simulink model "unityVPC"  (R2021a)
settings: Solver=FixedStepAuto  StartTime=0.0  StopTime=inf  FixedStep=0.02  RelTol=1e-3
undefined symbols (not defined in the file): alpha, Angular, gd, Kc, Linear, ros_freq, Rx, Ry, Rz, T, var_max, X, Y, Z
libraries: simlib_vpc_coremath x26, robotlib x20, simlib_vpc_basic x10, dspmtrx3 x4, simlib_vpc_gp x3
settings Model: EnablePacing=on  OrderedModelArguments=off  Creator=marco  LastModifiedBy=marco
settings DebuggingCC: AlgebraicLoopMsg=none

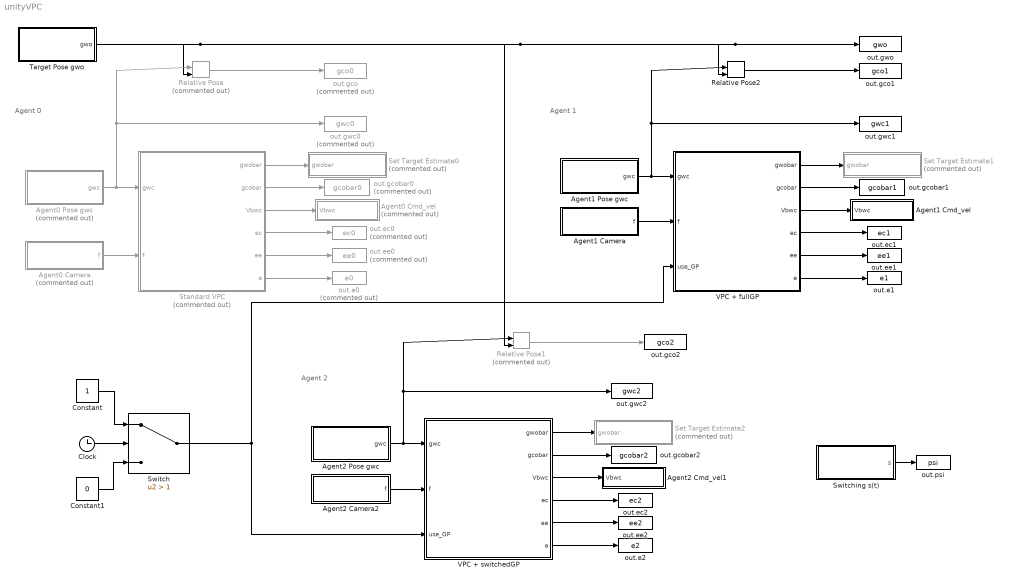
== system unityVPC ==
  note: Agent 0
  note: Agent 1
  note: Agent 2
  Agent0 Camera : Subsystem  Commented=on
  Agent0 Cmd_vel : Subsystem  Commented=on
  Agent0 Pose gwc : Subsystem  Commented=on
  Agent1 Camera : Subsystem
  Agent1 Cmd_vel : Subsystem
  Agent1 Pose gwc : Subsystem
  Agent2 Camera2 : Subsystem
  Agent2 Cmd_vel1 : Subsystem
  Agent2 Pose gwc : Subsystem
  Clock : Clock
  Constant : Constant
  Constant1 : Constant  Value=0
  Relative Pose : simlib_vpc_coremath/Relative Pose  Commented=on
      settings: SourceProductName=VPC Library
  Relative Pose1 : simlib_vpc_coremath/Relative Pose  Commented=on
      settings: SourceProductName=VPC Library
  Relative Pose2 : simlib_vpc_coremath/Relative Pose
      settings: SourceProductName=VPC Library
  Set Target Estimate0 : Subsystem  Commented=on
  Set Target Estimate1 : Subsystem  Commented=on
  Set Target Estimate2 : Subsystem  Commented=on
  Standard VPC : Subsystem  Commented=on
      mask Display:
      | disp('VPC without GP','texmode','on')
      | 
      | % Label ports
      | port_label('input',1,'g_{wc}','texmode','on')
      | port_label('input',2,'f','texmode','on')
      | port_label('output',1,'g_{wo,bar}','texmode','on')
      | port_label('output',2,'gco,bar','texmode','on')
      | port_label('output',3,'V^b_{wc}','texmode','on')
      | port_label('output',4,'ec','texmode','on')
      | port_label('output',5,'ee','texmode','on')
      | port_label('output',6,'e','texmode','on')
  Switch : Switch  Criteria=u2 > Threshold  Threshold=1
  Switching s(t) : Subsystem
  Target Pose gwo : Subsystem
  VPC + fullGP : Subsystem
      mask Display:
      | disp('VPC + fullGP','texmode','on')
      | 
      | % Label ports
      | port_label('input',1,'g_{wc}','texmode','on')
      | port_label('input',2,'f','texmode','on')
      | port_label('output',1,'g_{wo,bar}','texmode','on')
      | port_label('output',2,'gco,bar','texmode','on')
      | port_label('output',3,'V^b_{wc}','texmode','on')
      | port_label('output',4,'ec','texmode','on')
      | port_label('output',5,'ee','texmode','on')
      | port_label('output',6,'e','texmode','on')
  VPC + switchedGP : Subsystem
      mask Display:
      | disp('VPC + switchedGP','texmode','on')
      | 
      | % Label ports
      | port_label('input',1,'g_{wc}','texmode','on')
      | port_label('input',2,'f','texmode','on')
      | port_label('output',1,'g_{wo,bar}','texmode','on')
      | port_label('output',2,'gco,bar','texmode','on')
      | port_label('output',3,'V^b_{wc}','texmode','on')
      | port_label('output',4,'ec','texmode','on')
      | port_label('output',5,'ee','texmode','on')
      | port_label('output',6,'e','texmode','on')
  out.e0 : ToWorkspace  Commented=on  VariableName=e0  SaveFormat=Structure With Time  SampleTime=-1
  out.e1 : ToWorkspace  VariableName=e1  SaveFormat=Structure With Time  SampleTime=-1
  out.e2 : ToWorkspace  VariableName=e2  SaveFormat=Structure With Time  SampleTime=-1
  out.ec0 : ToWorkspace  Commented=on  VariableName=ec0  SaveFormat=Structure With Time  SampleTime=-1
  out.ec1 : ToWorkspace  VariableName=ec1  SaveFormat=Structure With Time  SampleTime=-1
  out.ec2 : ToWorkspace  VariableName=ec2  SaveFormat=Structure With Time  SampleTime=-1
  out.ee0 : ToWorkspace  Commented=on  VariableName=ee0  SaveFormat=Structure With Time  SampleTime=-1
  out.ee1 : ToWorkspace  VariableName=ee1  SaveFormat=Structure With Time  SampleTime=-1
  out.ee2 : ToWorkspace  VariableName=ee2  SaveFormat=Structure With Time  SampleTime=-1
  out.gco : ToWorkspace  Commented=on  VariableName=gco0  SaveFormat=Structure With Time  SampleTime=-1
  out.gco1 : ToWorkspace  VariableName=gco1  SaveFormat=Structure With Time  SampleTime=-1
  out.gco2 : ToWorkspace  VariableName=gco2  SaveFormat=Structure With Time  SampleTime=-1
  out.gcobar0 : ToWorkspace  Commented=on  VariableName=gcobar0  SaveFormat=Structure With Time  SampleTime=-1
  out.gcobar1 : ToWorkspace  VariableName=gcobar1  SaveFormat=Structure With Time  SampleTime=-1
  out.gcobar2 : ToWorkspace  VariableName=gcobar2  SaveFormat=Structure With Time  SampleTime=-1
  out.gwc0 : ToWorkspace  Commented=on  VariableName=gwc0  SaveFormat=Structure With Time  SampleTime=-1
  out.gwc1 : ToWorkspace  VariableName=gwc1  SaveFormat=Structure With Time  SampleTime=-1
  out.gwc2 : ToWorkspace  VariableName=gwc2  SaveFormat=Structure With Time  SampleTime=-1
  out.gwo : ToWorkspace  VariableName=gwo  SaveFormat=Structure With Time  SampleTime=-1
  out.psi : ToWorkspace  VariableName=psi  SaveFormat=Structure With Time  SampleTime=-1
  wires:
  Standard VPC/1(gwobar) -> Set Target Estimate0/1(gwobar)
  Agent0 Camera/1(f) -> Standard VPC/2(f)
  Relative Pose/1 -> out.gco/1
  Target Pose gwo/1(gwo) -> out.gwo/1, Relative Pose2/2, Relative Pose1/2, Relative Pose/2
  Agent0 Pose gwc/1(gwc) -> Relative Pose/1, out.gwc0/1, Standard VPC/1(gwc)
  Standard VPC/4(ec) -> out.ec0/1
  Standard VPC/5(ee) -> out.ee0/1
  Standard VPC/6(e) -> out.e0/1
  Standard VPC/2(gcobar) -> out.gcobar0/1
  Standard VPC/3(Vbwc) -> Agent0 Cmd_vel/1(Vbwc)
  Relative Pose1/1 -> out.gco2/1
  VPC + fullGP/4(ec) -> out.ec1/1
  VPC + fullGP/2(gcobar) -> out.gcobar1/1
  VPC + fullGP/5(ee) -> out.ee1/1
  VPC + fullGP/3(Vbwc) -> Agent1 Cmd_vel/1(Vbwc)
  Agent1 Pose gwc/1(gwc) -> Relative Pose2/1, out.gwc1/1, VPC + fullGP/1(gwc)
  VPC + fullGP/1(gwobar) -> Set Target Estimate1/1(gwobar)
  VPC + fullGP/6(e) -> out.e1/1
  Agent1 Camera/1(f) -> VPC + fullGP/2(f)
  Relative Pose2/1 -> out.gco1/1
  VPC + switchedGP/4(ec) -> out.ec2/1
  Agent2 Pose gwc/1(gwc) -> Relative Pose1/1, out.gwc2/1, VPC + switchedGP/1(gwc)
  VPC + switchedGP/2(gcobar) -> out.gcobar2/1
  Agent2 Camera2/1(f) -> VPC + switchedGP/2(f)
  VPC + switchedGP/5(ee) -> out.ee2/1
  VPC + switchedGP/1(gwobar) -> Set Target Estimate2/1(gwobar)
  VPC + switchedGP/3(Vbwc) -> Agent2 Cmd_vel1/1(Vbwc)
  VPC + switchedGP/6(e) -> out.e2/1
  Switching s(t)/1(s) -> out.psi/1
  Constant/1 -> Switch/1
  Constant1/1 -> Switch/3
  Switch/1 -> VPC + switchedGP/3(use_GP), VPC + fullGP/3(use_GP)
  Clock/1 -> Switch/2

== system unityVPC/Agent0 Camera ==
  Bus Selector1 : BusSelector  OutputSignals=Fp1X,Fp1Y,Fp2X,Fp2Y,Fp3X,Fp3Y,Fp4X,Fp4Y
  Data Type Conversion : DataTypeConversion  OutDataTypeStr=double
  Subscribe1 : robotlib/Subscribe  topicSource=Specify your own  topic=/agent0_vcam  messageType=custom_msgs/VisMea  SampleTime=-1  legacyBusStruct=off  messageQueueLength=1
  Terminator1 : Terminator
  Vector Concatenate : Concatenate  NumInputs=8
  f : Outport
  wires:
  Bus Selector1/4 -> Vector Concatenate/4  "<Fp2Y>"
  Data Type Conversion/1 -> f/1
  Bus Selector1/2 -> Vector Concatenate/2  "<Fp1Y>"
  Bus Selector1/3 -> Vector Concatenate/3  "<Fp2X>"
  Vector Concatenate/1 -> Data Type Conversion/1
  Subscribe1/1 -> Terminator1/1
  Bus Selector1/5 -> Vector Concatenate/5  "<Fp3X>"
  Bus Selector1/1 -> Vector Concatenate/1  "<Fp1X>"
  Subscribe1/2 -> Bus Selector1/1
  Bus Selector1/7 -> Vector Concatenate/7  "<Fp4X>"
  Bus Selector1/6 -> Vector Concatenate/6  "<Fp3Y>"
  Bus Selector1/8 -> Vector Concatenate/8  "<Fp4Y>"

== system unityVPC/Agent0 Cmd_vel ==
  note: Update estimate in Unity simulation
  Vbwc : Inport
  Blank Message : robotlib/Blank Message  messageClass=Message  entityType=geometry_msgs/Twist  messageType=geometry_msgs/Twist  SampleTime=inf  legacyBusStruct=off
  Bus Assignment1 : BusAssignment  AssignedSignals=Linear.X,Linear.Y,Linear.Z,Angular.X,Angular.Y,Angular.Z
  Demux1 : Demux  Outputs=6
  Gain : Gain  Gain=-1
  Gain1 : Gain  Gain=-1
  Gain2 : Gain  Gain=-1
  Publish : robotlib/Publish  topicSource=Specify your own  topic=/agent0_Vbwc  messageType=geometry_msgs/Twist  legacyBusStruct=off  messageQueueLength=1
  Rate Transition : RateTransition  Commented=through  OutPortSampleTime=1/ros_freq
  wires:
  Blank Message/1 -> Bus Assignment1/1
  Bus Assignment1/1 -> Publish/1
  Demux1/1 -> Bus Assignment1/2
  Demux1/4 -> Gain/1
  Vbwc/1 -> Rate Transition/1
  Demux1/5 -> Gain2/1
  Demux1/2 -> Bus Assignment1/4
  Demux1/3 -> Bus Assignment1/3
  Demux1/6 -> Gain1/1
  Gain/1 -> Bus Assignment1/5
  Gain1/1 -> Bus Assignment1/6
  Gain2/1 -> Bus Assignment1/7
  Rate Transition/1 -> Demux1/1

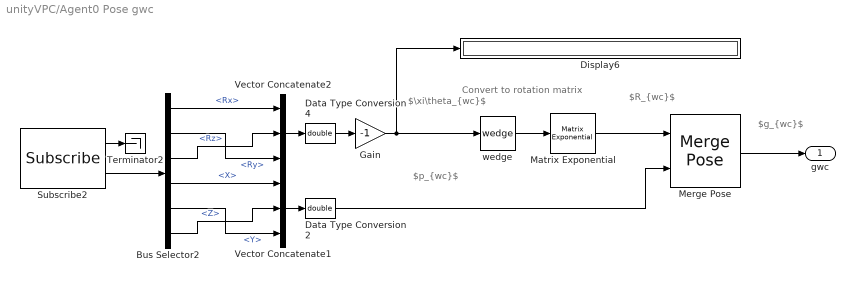
== system unityVPC/Agent0 Pose gwc ==
  note: $g_{wc}$
  note: $R_{wc}$
  note: $p_{wc}$
  note: $\xi\theta_{wc}$
  note: Convert to rotation matrix
  Bus Selector2 : BusSelector  OutputSignals=Rx,Ry,Rz,X,Y,Z
  Data Type Conversion2 : DataTypeConversion  OutDataTypeStr=double
  Data Type Conversion4 : DataTypeConversion  OutDataTypeStr=double
  Display6 : Display
  Gain : Gain  Gain=-1
  Matrix Exponential : dspmtrx3/Matrix Exponential
      settings: SourceProductBaseCode=DS
  Merge Pose : simlib_vpc_coremath/Merge Pose
      settings: SourceProductName=VPC Library
  Subscribe2 : robotlib/Subscribe  topicSource=Specify your own  topic=/agent0_pose  messageType=custom_msgs/PosRot  SampleTime=-1  legacyBusStruct=off  messageQueueLength=1
  Terminator2 : Terminator
  Vector Concatenate1 : Concatenate  NumInputs=3
  Vector Concatenate2 : Concatenate  NumInputs=3
  wedge : simlib_vpc_coremath/wedge
      settings: SourceProductName=VPC Library
  gwc : Outport
  wires:
  Vector Concatenate2/1 -> Data Type Conversion4/1
  Subscribe2/1 -> Terminator2/1
  Matrix Exponential/1 -> Merge Pose/1
  Vector Concatenate1/1 -> Data Type Conversion2/1
  Data Type Conversion2/1 -> Merge Pose/2
  Subscribe2/2 -> Bus Selector2/1
  Bus Selector2/1 -> Vector Concatenate2/1  "<Rx>"
  Bus Selector2/4 -> Vector Concatenate1/1  "<X>"
  Data Type Conversion4/1 -> Gain/1
  wedge/1 -> Matrix Exponential/1
  Bus Selector2/2 -> Vector Concatenate2/3  "<Ry>"
  Merge Pose/1 -> gwc/1
  Bus Selector2/5 -> Vector Concatenate1/3  "<Y>"
  Bus Selector2/6 -> Vector Concatenate1/2  "<Z>"
  Bus Selector2/3 -> Vector Concatenate2/2  "<Rz>"
  Gain/1 -> Display6/1, wedge/1

== system unityVPC/Agent1 Camera ==
  Bus Selector1 : BusSelector  OutputSignals=Fp1X,Fp1Y,Fp2X,Fp2Y,Fp3X,Fp3Y,Fp4X,Fp4Y
  Data Type Conversion : DataTypeConversion  OutDataTypeStr=double
  Subscribe1 : robotlib/Subscribe  topicSource=Select from ROS network  topic=/agent1_vcam  messageType=custom_msgs/VisMea  SampleTime=-1  legacyBusStruct=off  messageQueueLength=1
  Terminator1 : Terminator
  Vector Concatenate : Concatenate  NumInputs=8
  f : Outport
  wires:
  Bus Selector1/4 -> Vector Concatenate/4  "<Fp2Y>"
  Data Type Conversion/1 -> f/1
  Bus Selector1/2 -> Vector Concatenate/2  "<Fp1Y>"
  Bus Selector1/3 -> Vector Concatenate/3  "<Fp2X>"
  Vector Concatenate/1 -> Data Type Conversion/1
  Subscribe1/1 -> Terminator1/1
  Bus Selector1/5 -> Vector Concatenate/5  "<Fp3X>"
  Bus Selector1/1 -> Vector Concatenate/1  "<Fp1X>"
  Subscribe1/2 -> Bus Selector1/1
  Bus Selector1/7 -> Vector Concatenate/7  "<Fp4X>"
  Bus Selector1/6 -> Vector Concatenate/6  "<Fp3Y>"
  Bus Selector1/8 -> Vector Concatenate/8  "<Fp4Y>"

== system unityVPC/Agent1 Cmd_vel ==
  note: Update estimate in Unity simulation
  Vbwc : Inport
  Blank Message : robotlib/Blank Message  messageClass=Message  entityType=geometry_msgs/Twist  messageType=geometry_msgs/Twist  SampleTime=inf  legacyBusStruct=off
  Bus Assignment1 : BusAssignment  AssignedSignals=Linear.X,Linear.Y,Linear.Z,Angular.X,Angular.Y,Angular.Z
  Demux1 : Demux  Outputs=6
  Gain : Gain  Gain=-1
  Gain1 : Gain  Gain=-1
  Gain2 : Gain  Gain=-1
  Publish : robotlib/Publish  topicSource=Select from ROS network  topic=/agent1_Vbwc  messageType=geometry_msgs/Twist  legacyBusStruct=off  messageQueueLength=1
  Rate Transition : RateTransition  OutPortSampleTime=1/ros_freq
  wires:
  Blank Message/1 -> Bus Assignment1/1
  Bus Assignment1/1 -> Publish/1
  Demux1/1 -> Bus Assignment1/2
  Demux1/4 -> Gain/1
  Vbwc/1 -> Rate Transition/1
  Demux1/5 -> Gain2/1
  Demux1/2 -> Bus Assignment1/4
  Demux1/3 -> Bus Assignment1/3
  Demux1/6 -> Gain1/1
  Gain/1 -> Bus Assignment1/5
  Gain1/1 -> Bus Assignment1/6
  Gain2/1 -> Bus Assignment1/7
  Rate Transition/1 -> Demux1/1

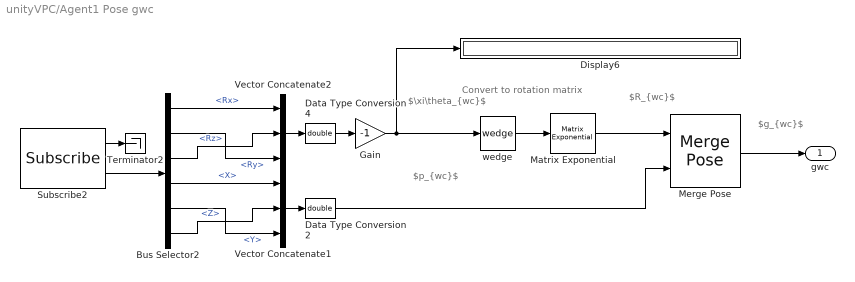
== system unityVPC/Agent1 Pose gwc ==
  note: $g_{wc}$
  note: $R_{wc}$
  note: $p_{wc}$
  note: $\xi\theta_{wc}$
  note: Convert to rotation matrix
  Bus Selector2 : BusSelector  OutputSignals=Rx,Ry,Rz,X,Y,Z
  Data Type Conversion2 : DataTypeConversion  OutDataTypeStr=double
  Data Type Conversion4 : DataTypeConversion  OutDataTypeStr=double
  Display6 : Display
  Gain : Gain  Gain=-1
  Matrix Exponential : dspmtrx3/Matrix Exponential
      settings: SourceProductBaseCode=DS
  Merge Pose : simlib_vpc_coremath/Merge Pose
      settings: SourceProductName=VPC Library
  Subscribe2 : robotlib/Subscribe  topicSource=Select from ROS network  topic=/agent1_pose  messageType=custom_msgs/PosRot  SampleTime=-1  legacyBusStruct=off  messageQueueLength=1
  Terminator2 : Terminator
  Vector Concatenate1 : Concatenate  NumInputs=3
  Vector Concatenate2 : Concatenate  NumInputs=3
  wedge : simlib_vpc_coremath/wedge
      settings: SourceProductName=VPC Library
  gwc : Outport
  wires:
  Vector Concatenate2/1 -> Data Type Conversion4/1
  Subscribe2/1 -> Terminator2/1
  Matrix Exponential/1 -> Merge Pose/1
  Vector Concatenate1/1 -> Data Type Conversion2/1
  Data Type Conversion2/1 -> Merge Pose/2
  Subscribe2/2 -> Bus Selector2/1
  Bus Selector2/1 -> Vector Concatenate2/1  "<Rx>"
  Bus Selector2/4 -> Vector Concatenate1/1  "<X>"
  Data Type Conversion4/1 -> Gain/1
  wedge/1 -> Matrix Exponential/1
  Bus Selector2/2 -> Vector Concatenate2/3  "<Ry>"
  Merge Pose/1 -> gwc/1
  Bus Selector2/5 -> Vector Concatenate1/3  "<Y>"
  Bus Selector2/6 -> Vector Concatenate1/2  "<Z>"
  Bus Selector2/3 -> Vector Concatenate2/2  "<Rz>"
  Gain/1 -> Display6/1, wedge/1

== system unityVPC/Agent2 Camera2 ==
  Bus Selector1 : BusSelector  OutputSignals=Fp1X,Fp1Y,Fp2X,Fp2Y,Fp3X,Fp3Y,Fp4X,Fp4Y
  Data Type Conversion : DataTypeConversion  OutDataTypeStr=double
  Subscribe1 : robotlib/Subscribe  topicSource=Specify your own  topic=/agent2_vcam  messageType=custom_msgs/VisMea  SampleTime=-1  legacyBusStruct=off  messageQueueLength=1
  Terminator1 : Terminator
  Vector Concatenate : Concatenate  NumInputs=8
  f : Outport
  wires:
  Bus Selector1/4 -> Vector Concatenate/4  "<Fp2Y>"
  Data Type Conversion/1 -> f/1
  Bus Selector1/2 -> Vector Concatenate/2  "<Fp1Y>"
  Bus Selector1/3 -> Vector Concatenate/3  "<Fp2X>"
  Vector Concatenate/1 -> Data Type Conversion/1
  Subscribe1/1 -> Terminator1/1
  Bus Selector1/5 -> Vector Concatenate/5  "<Fp3X>"
  Bus Selector1/1 -> Vector Concatenate/1  "<Fp1X>"
  Subscribe1/2 -> Bus Selector1/1
  Bus Selector1/7 -> Vector Concatenate/7  "<Fp4X>"
  Bus Selector1/6 -> Vector Concatenate/6  "<Fp3Y>"
  Bus Selector1/8 -> Vector Concatenate/8  "<Fp4Y>"

== system unityVPC/Agent2 Cmd_vel1 ==
  note: Update estimate in Unity simulation
  Vbwc : Inport
  Blank Message : robotlib/Blank Message  messageClass=Message  entityType=geometry_msgs/Twist  messageType=geometry_msgs/Twist  SampleTime=inf  legacyBusStruct=off
  Bus Assignment1 : BusAssignment  AssignedSignals=Linear.X,Linear.Y,Linear.Z,Angular.X,Angular.Y,Angular.Z
  Demux1 : Demux  Outputs=6
  Gain : Gain  Gain=-1
  Gain1 : Gain  Gain=-1
  Gain2 : Gain  Gain=-1
  Publish : robotlib/Publish  topicSource=Specify your own  topic=/agent2_Vbwc  messageType=geometry_msgs/Twist  legacyBusStruct=off  messageQueueLength=1
  Rate Transition : RateTransition  OutPortSampleTime=1/ros_freq
  wires:
  Blank Message/1 -> Bus Assignment1/1
  Bus Assignment1/1 -> Publish/1
  Demux1/1 -> Bus Assignment1/2
  Demux1/4 -> Gain/1
  Vbwc/1 -> Rate Transition/1
  Demux1/5 -> Gain2/1
  Demux1/2 -> Bus Assignment1/4
  Demux1/3 -> Bus Assignment1/3
  Demux1/6 -> Gain1/1
  Gain/1 -> Bus Assignment1/5
  Gain1/1 -> Bus Assignment1/6
  Gain2/1 -> Bus Assignment1/7
  Rate Transition/1 -> Demux1/1

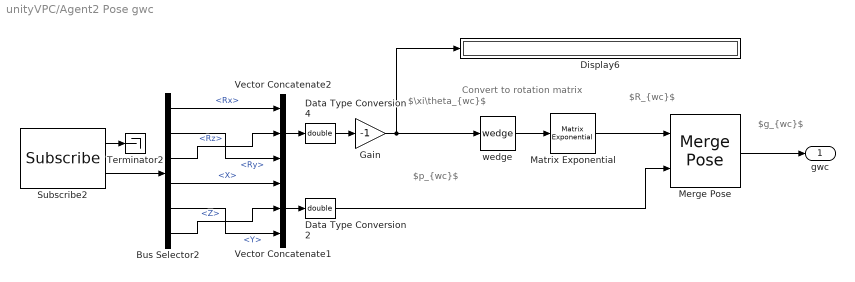
== system unityVPC/Agent2 Pose gwc ==
  note: $g_{wc}$
  note: $R_{wc}$
  note: $p_{wc}$
  note: $\xi\theta_{wc}$
  note: Convert to rotation matrix
  Bus Selector2 : BusSelector  OutputSignals=Rx,Ry,Rz,X,Y,Z
  Data Type Conversion2 : DataTypeConversion  OutDataTypeStr=double
  Data Type Conversion4 : DataTypeConversion  OutDataTypeStr=double
  Display6 : Display
  Gain : Gain  Gain=-1
  Matrix Exponential : dspmtrx3/Matrix Exponential
      settings: SourceProductBaseCode=DS
  Merge Pose : simlib_vpc_coremath/Merge Pose
      settings: SourceProductName=VPC Library
  Subscribe2 : robotlib/Subscribe  topicSource=Specify your own  topic=/agent2_pose  messageType=custom_msgs/PosRot  SampleTime=-1  legacyBusStruct=off  messageQueueLength=1
  Terminator2 : Terminator
  Vector Concatenate1 : Concatenate  NumInputs=3
  Vector Concatenate2 : Concatenate  NumInputs=3
  wedge : simlib_vpc_coremath/wedge
      settings: SourceProductName=VPC Library
  gwc : Outport
  wires:
  Vector Concatenate2/1 -> Data Type Conversion4/1
  Subscribe2/1 -> Terminator2/1
  Matrix Exponential/1 -> Merge Pose/1
  Vector Concatenate1/1 -> Data Type Conversion2/1
  Data Type Conversion2/1 -> Merge Pose/2
  Subscribe2/2 -> Bus Selector2/1
  Bus Selector2/1 -> Vector Concatenate2/1  "<Rx>"
  Bus Selector2/4 -> Vector Concatenate1/1  "<X>"
  Data Type Conversion4/1 -> Gain/1
  wedge/1 -> Matrix Exponential/1
  Bus Selector2/2 -> Vector Concatenate2/3  "<Ry>"
  Merge Pose/1 -> gwc/1
  Bus Selector2/5 -> Vector Concatenate1/3  "<Y>"
  Bus Selector2/6 -> Vector Concatenate1/2  "<Z>"
  Bus Selector2/3 -> Vector Concatenate2/2  "<Rz>"
  Gain/1 -> Display6/1, wedge/1

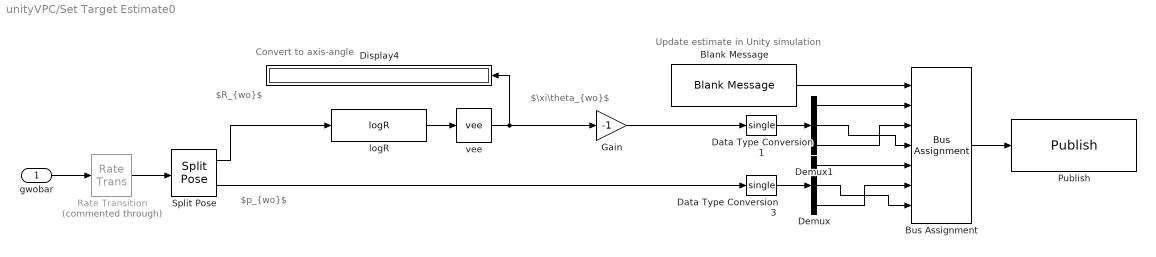
== system unityVPC/Set Target Estimate0 ==
  note: $\xi\theta_{wo}$
  note: $p_{wo}$
  note: Convert to axis-angle
  note: $R_{wo}$
  note: Update estimate in Unity simulation
  gwobar : Inport
  Blank Message : robotlib/Blank Message  messageClass=Message  entityType=custom_msgs/PosRot  messageType=custom_msgs/PosRot  SampleTime=inf  legacyBusStruct=off
  Bus Assignment : BusAssignment  AssignedSignals=Rx,Ry,Rz,X,Y,Z
  Data Type Conversion1 : DataTypeConversion  OutDataTypeStr=single
  Data Type Conversion3 : DataTypeConversion  OutDataTypeStr=single
  Demux : Demux  Outputs=3
  Demux1 : Demux  Outputs=3
  Display4 : Display
  Gain : Gain  Gain=-1
  Publish : robotlib/Publish  topicSource=Select from ROS network  topic=/estim_pose  messageType=custom_msgs/PosRot  legacyBusStruct=off  messageQueueLength=1
  Rate Transition : RateTransition  Commented=through  OutPortSampleTime=1/ros_freq
  Split Pose : simlib_vpc_coremath/Split Pose
      settings: SourceProductName=VPC Library
  logR : simlib_vpc_coremath/logR
      settings: SourceProductName=VPC Library
  vee : simlib_vpc_coremath/vee
      settings: SourceProductName=VPC Library
  wires:
  Bus Assignment/1 -> Publish/1
  Demux1/1 -> Bus Assignment/2
  Data Type Conversion1/1 -> Demux1/1
  Demux1/2 -> Bus Assignment/4
  vee/1 -> Gain/1, Display4/1
  Split Pose/1 -> logR/1
  Demux/3 -> Bus Assignment/6
  Blank Message/1 -> Bus Assignment/1
  Demux1/3 -> Bus Assignment/3
  Split Pose/2 -> Data Type Conversion3/1
  Demux/1 -> Bus Assignment/5
  logR/1 -> vee/1
  Data Type Conversion3/1 -> Demux/1
  Demux/2 -> Bus Assignment/7
  gwobar/1 -> Rate Transition/1
  Gain/1 -> Data Type Conversion1/1
  Rate Transition/1 -> Split Pose/1

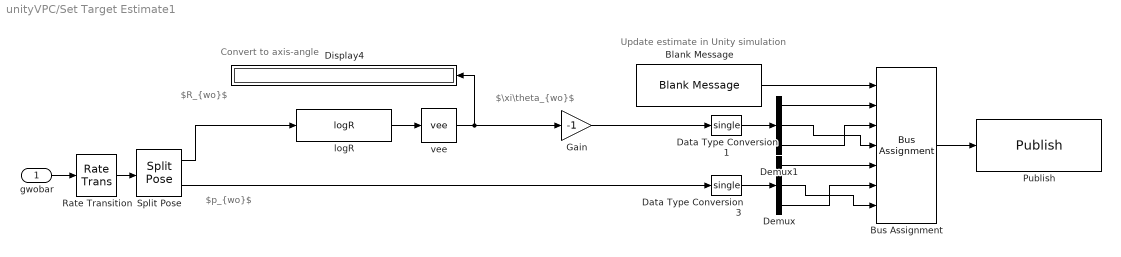
== system unityVPC/Set Target Estimate1 ==
  note: $\xi\theta_{wo}$
  note: $p_{wo}$
  note: Convert to axis-angle
  note: $R_{wo}$
  note: Update estimate in Unity simulation
  gwobar : Inport
  Blank Message : robotlib/Blank Message  messageClass=Message  entityType=custom_msgs/PosRot  messageType=custom_msgs/PosRot  SampleTime=inf  legacyBusStruct=off
  Bus Assignment : BusAssignment  AssignedSignals=Rx,Ry,Rz,X,Y,Z
  Data Type Conversion1 : DataTypeConversion  OutDataTypeStr=single
  Data Type Conversion3 : DataTypeConversion  OutDataTypeStr=single
  Demux : Demux  Outputs=3
  Demux1 : Demux  Outputs=3
  Display4 : Display
  Gain : Gain  Gain=-1
  Publish : robotlib/Publish  topicSource=Select from ROS network  topic=/estim_pose  messageType=custom_msgs/PosRot  legacyBusStruct=off  messageQueueLength=1
  Rate Transition : RateTransition  OutPortSampleTime=1/ros_freq
  Split Pose : simlib_vpc_coremath/Split Pose
      settings: SourceProductName=VPC Library
  logR : simlib_vpc_coremath/logR
      settings: SourceProductName=VPC Library
  vee : simlib_vpc_coremath/vee
      settings: SourceProductName=VPC Library
  wires:
  Bus Assignment/1 -> Publish/1
  Demux1/1 -> Bus Assignment/2
  Data Type Conversion1/1 -> Demux1/1
  Demux1/2 -> Bus Assignment/4
  vee/1 -> Gain/1, Display4/1
  Split Pose/1 -> logR/1
  Demux/3 -> Bus Assignment/6
  Blank Message/1 -> Bus Assignment/1
  Demux1/3 -> Bus Assignment/3
  Split Pose/2 -> Data Type Conversion3/1
  Demux/1 -> Bus Assignment/5
  logR/1 -> vee/1
  Data Type Conversion3/1 -> Demux/1
  Demux/2 -> Bus Assignment/7
  gwobar/1 -> Rate Transition/1
  Gain/1 -> Data Type Conversion1/1
  Rate Transition/1 -> Split Pose/1

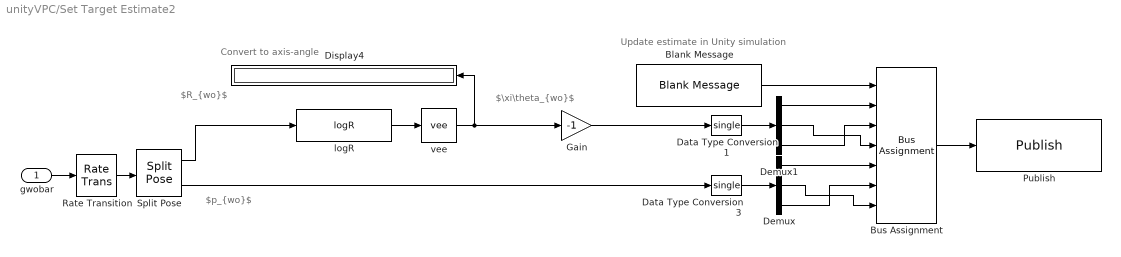
== system unityVPC/Set Target Estimate2 ==
  note: $\xi\theta_{wo}$
  note: $p_{wo}$
  note: Convert to axis-angle
  note: $R_{wo}$
  note: Update estimate in Unity simulation
  gwobar : Inport
  Blank Message : robotlib/Blank Message  messageClass=Message  entityType=custom_msgs/PosRot  messageType=custom_msgs/PosRot  SampleTime=inf  legacyBusStruct=off
  Bus Assignment : BusAssignment  AssignedSignals=Rx,Ry,Rz,X,Y,Z
  Data Type Conversion1 : DataTypeConversion  OutDataTypeStr=single
  Data Type Conversion3 : DataTypeConversion  OutDataTypeStr=single
  Demux : Demux  Outputs=3
  Demux1 : Demux  Outputs=3
  Display4 : Display
  Gain : Gain  Gain=-1
  Publish : robotlib/Publish  topicSource=Select from ROS network  topic=/estim_pose  messageType=custom_msgs/PosRot  legacyBusStruct=off  messageQueueLength=1
  Rate Transition : RateTransition  OutPortSampleTime=1/ros_freq
  Split Pose : simlib_vpc_coremath/Split Pose
      settings: SourceProductName=VPC Library
  logR : simlib_vpc_coremath/logR
      settings: SourceProductName=VPC Library
  vee : simlib_vpc_coremath/vee
      settings: SourceProductName=VPC Library
  wires:
  Bus Assignment/1 -> Publish/1
  Demux1/1 -> Bus Assignment/2
  Data Type Conversion1/1 -> Demux1/1
  Demux1/2 -> Bus Assignment/4
  vee/1 -> Gain/1, Display4/1
  Split Pose/1 -> logR/1
  Demux/3 -> Bus Assignment/6
  Blank Message/1 -> Bus Assignment/1
  Demux1/3 -> Bus Assignment/3
  Split Pose/2 -> Data Type Conversion3/1
  Demux/1 -> Bus Assignment/5
  logR/1 -> vee/1
  Data Type Conversion3/1 -> Demux/1
  Demux/2 -> Bus Assignment/7
  gwobar/1 -> Rate Transition/1
  Gain/1 -> Data Type Conversion1/1
  Rate Transition/1 -> Split Pose/1

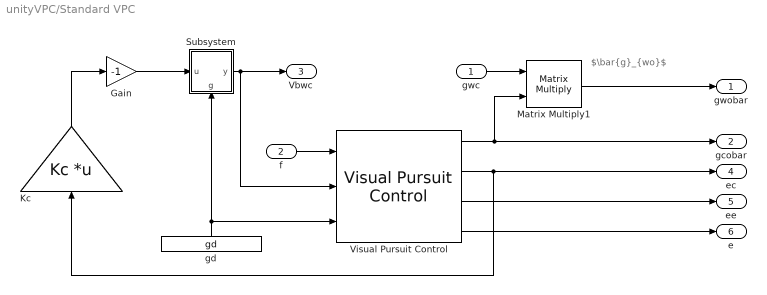
== system unityVPC/Standard VPC ==
  note: $\bar{g}_{wo}$
  gwc : Inport
  f : Inport  Port=2
  Gain : Gain  Gain=-1
  Kc : Gain  Gain=Kc  Multiplication=Matrix(K*u) (u vector)
  Matrix Multiply1 : Product  Multiplication=Matrix(*)
  Subsystem : Subsystem
      settings: PortSchema="{\"entries\":[{\"content\":{\"sides\":[{\"content\":{\"connectorIds\":[\"In1\"]},\"type\":\"ConnectorPlacement.EquallySpacedRectSide\",\"uuid\":\"72e68008-5c4a-43a9-a560-64c6a31a0c08\"},{\"content\":{\"connectorIds\":[\"Out1\"],\"side\":\"RIGHT\"},\"type\":\"ConnectorPlacement.EquallySpacedRectSide\",\"uuid\":\"da07f5ff-2b2c-4c55-a2f2-34e133777503\"},{\"content\":{\"connectorIds\":[],\"side\":\"TOP\"},\"type\":\"ConnectorPlacement.EquallySpacedRectSide\",\"uuid\":\"6d174428-4364-4e89-aba7-4e9864808ab5\"},{\"content\":{\"connectorIds\":[\"In2\"],\"side\":\"BOTTOM\"},\"type\":\"ConnectorPlacement.EquallySpacedRectSide\",\"uuid\":\"f9633104-9c11-4d21-90a7-e0f886d9e92d\"},{\"content\":{\"connectorIds\":[],\"side\":\"HIDDEN\"},\"type\":\"ConnectorPlacement.EquallySpacedRectSide\",\"uuid\":\"662f08ae-9279-4a4f-85ea-81d97ead27d9\"}]},\"type\":\"ConnectorPlacement.EquallySpacedConnector\",\"uuid\":\"f3cd156c-cccd-47c6-b81c-6113f78efd58\"}],\"packageUris\":[\"http://schema.mathworks.com/mf0/Connector/R2020b\"],\"version\":\"1.0\"}"
      mask Display:
      | % Glitch in Matlab: If you define a line whose starting point and end point
      | % is equal, then the entire mask block is plotted in bold
      | plot([0,0],[0,0])
      | 
      | % Draw box
      | indent = 0.3;
      | ang=[0:0.2:pi/2, pi/2];
      | plot([0,1-indent],[0,0])
      | xp=indent*sin(ang)+1-indent;
      | yp=indent-indent*cos(ang);
      | plot(xp,yp);
      | plot([1,1,indent],[indent,1,1])
      | xp=indent-indent*sin(ang);
      | yp=1-indent+indent*cos(ang);
      | plot(xp,yp);
      | plot([0,0],[1-indent,0])
      | 
      | % Write label & ports
      | disp('-Ad_{(g_d)}','texmode','on')
      | text(0.5,0.2,'\fontsize{7}g_d','texmode','on')
  Visual Pursuit Control : simlib_vpc_basic/Visual Pursuit Control  gd_source=external  gd_value=[eye(4,3),ones(4,1)]  show_ee=on  show_e=on  show_nu=off  show_dgcobar=off  show_gce=off  gcobar0=gco_init  Ke_source=internal  Ke=Ke  show_ue_aux=off  projection=on  camtype=Pinhole  fo=fp  lambda=lambda
      settings: SourceProductName=VPC Library
  gd : Constant  Value=gd
  gwobar : Outport
  gcobar : Outport  Port=2
  Vbwc : Outport  Port=3
  ec : Outport  Port=4
  ee : Outport  Port=5
  e : Outport  Port=6
  wires:
  f/1 -> Visual Pursuit Control/1
  Matrix Multiply1/1 -> gwobar/1
  Subsystem/1(y) -> Vbwc/1, Visual Pursuit Control/2
  gwc/1 -> Matrix Multiply1/1
  Kc/1 -> Gain/1
  Visual Pursuit Control/4 -> e/1
  Gain/1 -> Subsystem/1(u)
  Visual Pursuit Control/2 -> ec/1, Kc/1
  Visual Pursuit Control/3 -> ee/1
  gd/1 -> Subsystem/2(g), Visual Pursuit Control/3
  Visual Pursuit Control/1 -> gcobar/1, Matrix Multiply1/2

== system unityVPC/Switching s(t) ==
  Bus Selector2 : BusSelector  OutputSignals=Data
  Data Type Conversion : DataTypeConversion  OutDataTypeStr=double
  Subscribe2 : robotlib/Subscribe  topicSource=Select from ROS network  topic=/switching  messageType=std_msgs/Int32  SampleTime=-1  legacyBusStruct=off  messageQueueLength=1
  Terminator2 : Terminator
  s : Outport
  wires:
  Subscribe2/1 -> Terminator2/1
  Subscribe2/2 -> Bus Selector2/1
  Bus Selector2/1 -> Data Type Conversion/1  "<Data>"
  Data Type Conversion/1 -> s/1

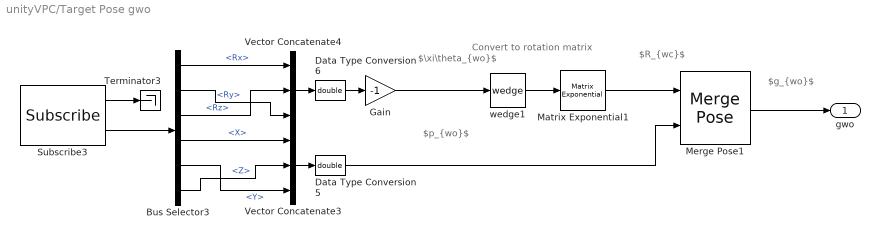
== system unityVPC/Target Pose gwo ==
  note: $\xi\theta_{wo}$
  note: Convert to rotation matrix
  note: $p_{wo}$
  note: $R_{wc}$
  note: $g_{wo}$
  Bus Selector3 : BusSelector  OutputSignals=Rx,Ry,Rz,X,Y,Z
  Data Type Conversion5 : DataTypeConversion  OutDataTypeStr=double
  Data Type Conversion6 : DataTypeConversion  OutDataTypeStr=double
  Gain : Gain  Gain=-1
  Matrix Exponential1 : dspmtrx3/Matrix Exponential
      settings: SourceProductBaseCode=DS
  Merge Pose1 : simlib_vpc_coremath/Merge Pose
      settings: SourceProductName=VPC Library
  Subscribe3 : robotlib/Subscribe  topicSource=Select from ROS network  topic=/target_pose  messageType=custom_msgs/PosRot  SampleTime=-1  legacyBusStruct=off  messageQueueLength=1
  Terminator3 : Terminator
  Vector Concatenate3 : Concatenate  NumInputs=3
  Vector Concatenate4 : Concatenate  NumInputs=3
  wedge1 : simlib_vpc_coremath/wedge
      settings: SourceProductName=VPC Library
  gwo : Outport
  wires:
  Data Type Conversion5/1 -> Merge Pose1/2
  Bus Selector3/4 -> Vector Concatenate3/1  "<X>"
  Vector Concatenate3/1 -> Data Type Conversion5/1
  wedge1/1 -> Matrix Exponential1/1
  Subscribe3/2 -> Bus Selector3/1
  Matrix Exponential1/1 -> Merge Pose1/1
  Vector Concatenate4/1 -> Data Type Conversion6/1
  Data Type Conversion6/1 -> Gain/1
  Bus Selector3/1 -> Vector Concatenate4/1  "<Rx>"
  Subscribe3/1 -> Terminator3/1
  Bus Selector3/3 -> Vector Concatenate4/2  "<Rz>"
  Bus Selector3/5 -> Vector Concatenate3/3  "<Y>"
  Bus Selector3/2 -> Vector Concatenate4/3  "<Ry>"
  Bus Selector3/6 -> Vector Concatenate3/2  "<Z>"
  Merge Pose1/1 -> gwo/1
  Gain/1 -> wedge1/1

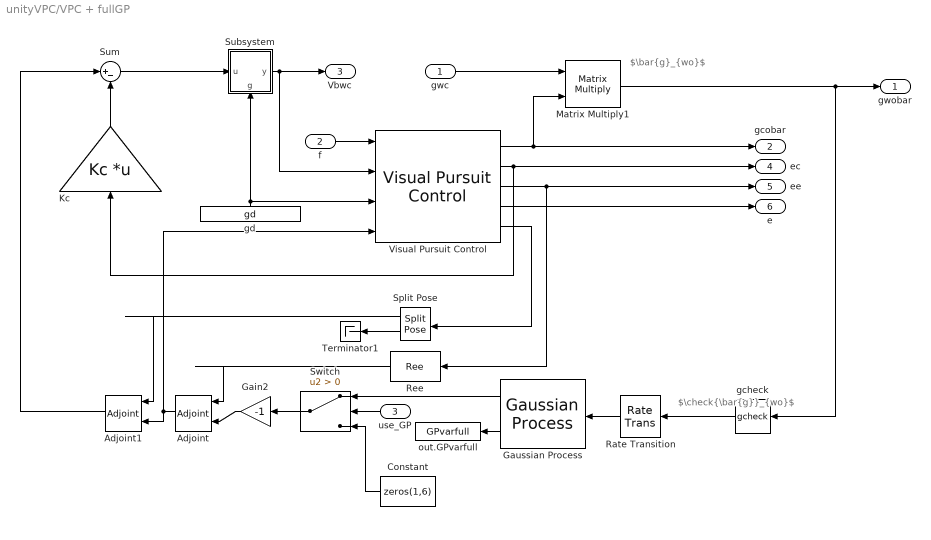
== system unityVPC/VPC + fullGP ==
  note: $\bar{g}_{wo}$
  note: $\check{\bar{g}}_{wo}$
  gwc : Inport
  f : Inport  Port=2
  use_GP : Inport  Port=3
  Adjoint : simlib_vpc_basic/Adjoint  adjointtype=orientation
      settings: SourceProductName=VPC Library
  Adjoint1 : simlib_vpc_basic/Adjoint  adjointtype=orientation
      settings: SourceProductName=VPC Library
  Constant : Constant  Value=zeros(1,6)
  Gain2 : Gain  Gain=-1
  Gaussian Process : simlib_vpc_gp/Gaussian Process  X=Xfull  Y=Yfull  sigman=snfull  kernel=Squared Exponential ARD  hyp=hypfull
      settings: SourceProductName=VPC Library
  Kc : Gain  Gain=Kc  Multiplication=Matrix(K*u) (u vector)
  Matrix Multiply1 : Product  Multiplication=Matrix(*)
  Rate Transition : RateTransition
  Ree : simlib_vpc_coremath/Ree
      settings: SourceProductName=VPC Library
  Split Pose : simlib_vpc_coremath/Split Pose
      settings: SourceProductName=VPC Library
  Subsystem : Subsystem
      settings: PortSchema="{\"entries\":[{\"content\":{\"sides\":[{\"content\":{\"connectorIds\":[\"In1\"]},\"type\":\"ConnectorPlacement.EquallySpacedRectSide\",\"uuid\":\"72e68008-5c4a-43a9-a560-64c6a31a0c08\"},{\"content\":{\"connectorIds\":[\"Out1\"],\"side\":\"RIGHT\"},\"type\":\"ConnectorPlacement.EquallySpacedRectSide\",\"uuid\":\"da07f5ff-2b2c-4c55-a2f2-34e133777503\"},{\"content\":{\"connectorIds\":[],\"side\":\"TOP\"},\"type\":\"ConnectorPlacement.EquallySpacedRectSide\",\"uuid\":\"6d174428-4364-4e89-aba7-4e9864808ab5\"},{\"content\":{\"connectorIds\":[\"In2\"],\"side\":\"BOTTOM\"},\"type\":\"ConnectorPlacement.EquallySpacedRectSide\",\"uuid\":\"f9633104-9c11-4d21-90a7-e0f886d9e92d\"},{\"content\":{\"connectorIds\":[],\"side\":\"HIDDEN\"},\"type\":\"ConnectorPlacement.EquallySpacedRectSide\",\"uuid\":\"662f08ae-9279-4a4f-85ea-81d97ead27d9\"}]},\"type\":\"ConnectorPlacement.EquallySpacedConnector\",\"uuid\":\"f3cd156c-cccd-47c6-b81c-6113f78efd58\"}],\"packageUris\":[\"http://schema.mathworks.com/mf0/Connector/R2020b\"],\"version\":\"1.0\"}"
      mask Display:
      | % Glitch in Matlab: If you define a line whose starting point and end point
      | % is equal, then the entire mask block is plotted in bold
      | plot([0,0],[0,0])
      | 
      | % Draw box
      | indent = 0.3;
      | ang=[0:0.2:pi/2, pi/2];
      | plot([0,1-indent],[0,0])
      | xp=indent*sin(ang)+1-indent;
      | yp=indent-indent*cos(ang);
      | plot(xp,yp);
      | plot([1,1,indent],[indent,1,1])
      | xp=indent-indent*sin(ang);
      | yp=1-indent+indent*cos(ang);
      | plot(xp,yp);
      | plot([0,0],[1-indent,0])
      | 
      | % Write label & ports
      | disp('-Ad_{(g_d)}','texmode','on')
      | text(0.5,0.2,'\fontsize{7}g_d','texmode','on')
  Sum : Sum  Inputs=|+-
  Switch : Switch  Criteria=u2 > Threshold
  Terminator1 : Terminator
  Visual Pursuit Control : simlib_vpc_basic/Visual Pursuit Control  gd_source=external  gd_value=[eye(4,3),ones(4,1)]  show_ee=on  show_e=on  show_nu=off  show_dgcobar=off  show_gce=on  gcobar0=gco_init  Ke_source=internal  Ke=Ke  show_ue_aux=on  projection=on  camtype=Pinhole  fo=fp  lambda=lambda
      settings: SourceProductName=VPC Library
  gcheck : simlib_vpc_coremath/gcheck
      settings: SourceProductName=VPC Library
  gd : Constant  Value=gd
  out.GPvarfull : ToWorkspace  VariableName=GPvarfull  SaveFormat=Structure With Time  SampleTime=-1
  gwobar : Outport
  gcobar : Outport  Port=2
  Vbwc : Outport  Port=3
  ec : Outport  Port=4
  ee : Outport  Port=5
  e : Outport  Port=6
  wires:
  f/1 -> Visual Pursuit Control/1
  Matrix Multiply1/1 -> gcheck/1, gwobar/1
  Subsystem/1(y) -> Vbwc/1, Visual Pursuit Control/2
  gwc/1 -> Matrix Multiply1/1
  Visual Pursuit Control/4 -> e/1
  Kc/1 -> Sum/2
  Visual Pursuit Control/2 -> ec/1, Kc/1
  Visual Pursuit Control/3 -> Ree/1, ee/1
  gd/1 -> Subsystem/2(g), Visual Pursuit Control/3
  Visual Pursuit Control/1 -> Matrix Multiply1/2, gcobar/1
  Split Pose/1 -> Adjoint1/2
  Rate Transition/1 -> Gaussian Process/1
  Adjoint/1 -> Visual Pursuit Control/4, Adjoint1/1
  Ree/1 -> Adjoint/2
  Split Pose/2 -> Terminator1/1
  Gain2/1 -> Adjoint/1
  Switch/1 -> Gain2/1
  Sum/1 -> Subsystem/1(u)
  Adjoint1/1 -> Sum/1
  Visual Pursuit Control/5 -> Split Pose/1
  Gaussian Process/2 -> out.GPvarfull/1
  gcheck/1 -> Rate Transition/1
  Gaussian Process/1 -> Switch/1
  Constant/1 -> Switch/3
  use_GP/1 -> Switch/2

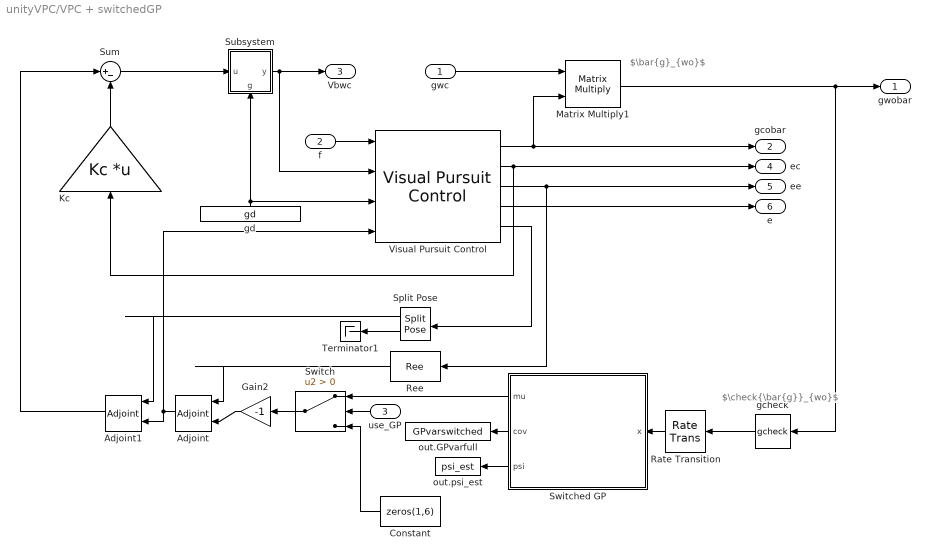
== system unityVPC/VPC + switchedGP ==
  note: $\bar{g}_{wo}$
  note: $\check{\bar{g}}_{wo}$
  gwc : Inport
  f : Inport  Port=2
  use_GP : Inport  Port=3
  Adjoint : simlib_vpc_basic/Adjoint  adjointtype=orientation
      settings: SourceProductName=VPC Library
  Adjoint1 : simlib_vpc_basic/Adjoint  adjointtype=orientation
      settings: SourceProductName=VPC Library
  Constant : Constant  Value=zeros(1,6)
  Gain2 : Gain  Gain=-1
  Kc : Gain  Gain=Kc  Multiplication=Matrix(K*u) (u vector)
  Matrix Multiply1 : Product  Multiplication=Matrix(*)
  Rate Transition : RateTransition
  Ree : simlib_vpc_coremath/Ree
      settings: SourceProductName=VPC Library
  Split Pose : simlib_vpc_coremath/Split Pose
      settings: SourceProductName=VPC Library
  Subsystem : Subsystem
      settings: PortSchema="{\"entries\":[{\"content\":{\"sides\":[{\"content\":{\"connectorIds\":[\"In1\"]},\"type\":\"ConnectorPlacement.EquallySpacedRectSide\",\"uuid\":\"72e68008-5c4a-43a9-a560-64c6a31a0c08\"},{\"content\":{\"connectorIds\":[\"Out1\"],\"side\":\"RIGHT\"},\"type\":\"ConnectorPlacement.EquallySpacedRectSide\",\"uuid\":\"da07f5ff-2b2c-4c55-a2f2-34e133777503\"},{\"content\":{\"connectorIds\":[],\"side\":\"TOP\"},\"type\":\"ConnectorPlacement.EquallySpacedRectSide\",\"uuid\":\"6d174428-4364-4e89-aba7-4e9864808ab5\"},{\"content\":{\"connectorIds\":[\"In2\"],\"side\":\"BOTTOM\"},\"type\":\"ConnectorPlacement.EquallySpacedRectSide\",\"uuid\":\"f9633104-9c11-4d21-90a7-e0f886d9e92d\"},{\"content\":{\"connectorIds\":[],\"side\":\"HIDDEN\"},\"type\":\"ConnectorPlacement.EquallySpacedRectSide\",\"uuid\":\"662f08ae-9279-4a4f-85ea-81d97ead27d9\"}]},\"type\":\"ConnectorPlacement.EquallySpacedConnector\",\"uuid\":\"f3cd156c-cccd-47c6-b81c-6113f78efd58\"}],\"packageUris\":[\"http://schema.mathworks.com/mf0/Connector/R2020b\"],\"version\":\"1.0\"}"
      mask Display:
      | % Glitch in Matlab: If you define a line whose starting point and end point
      | % is equal, then the entire mask block is plotted in bold
      | plot([0,0],[0,0])
      | 
      | % Draw box
      | indent = 0.3;
      | ang=[0:0.2:pi/2, pi/2];
      | plot([0,1-indent],[0,0])
      | xp=indent*sin(ang)+1-indent;
      | yp=indent-indent*cos(ang);
      | plot(xp,yp);
      | plot([1,1,indent],[indent,1,1])
      | xp=indent-indent*sin(ang);
      | yp=1-indent+indent*cos(ang);
      | plot(xp,yp);
      | plot([0,0],[1-indent,0])
      | 
      | % Write label & ports
      | disp('-Ad_{(g_d)}','texmode','on')
      | text(0.5,0.2,'\fontsize{7}g_d','texmode','on')
  Sum : Sum  Inputs=|+-
  Switch : Switch  Criteria=u2 > Threshold
  Switched GP : Subsystem
      mask Display:
      | disp('Switched GP','texmode','on')
      | 
      | % Label ports
      | port_label('input',1,'x*','texmode','on')
      | port_label('output',1,'\mu','texmode','on')
      | port_label('output',2,'\Sigma','texmode','on')
      | port_label('output',3,'\psi_{est}','texmode','on')
  Terminator1 : Terminator
  Visual Pursuit Control : simlib_vpc_basic/Visual Pursuit Control  gd_source=external  gd_value=[eye(4,3),ones(4,1)]  show_ee=on  show_e=on  show_nu=off  show_dgcobar=off  show_gce=on  gcobar0=gco_init  Ke_source=internal  Ke=Ke  show_ue_aux=on  projection=on  camtype=Pinhole  fo=fp  lambda=lambda
      settings: SourceProductName=VPC Library
  gcheck : simlib_vpc_coremath/gcheck
      settings: SourceProductName=VPC Library
  gd : Constant  Value=gd
  out.GPvarfull : ToWorkspace  VariableName=GPvarswitched  SaveFormat=Structure With Time  SampleTime=-1
  out.psi_est : ToWorkspace  VariableName=psi_est  SaveFormat=Structure With Time  SampleTime=-1
  gwobar : Outport
  gcobar : Outport  Port=2
  Vbwc : Outport  Port=3
  ec : Outport  Port=4
  ee : Outport  Port=5
  e : Outport  Port=6
  wires:
  f/1 -> Visual Pursuit Control/1
  Matrix Multiply1/1 -> gcheck/1, gwobar/1
  Subsystem/1(y) -> Vbwc/1, Visual Pursuit Control/2
  gwc/1 -> Matrix Multiply1/1
  Visual Pursuit Control/4 -> e/1
  Kc/1 -> Sum/2
  Visual Pursuit Control/2 -> ec/1, Kc/1
  Visual Pursuit Control/3 -> Ree/1, ee/1
  gd/1 -> Subsystem/2(g), Visual Pursuit Control/3
  Visual Pursuit Control/1 -> Matrix Multiply1/2, gcobar/1
  Split Pose/1 -> Adjoint1/2
  Adjoint/1 -> Visual Pursuit Control/4, Adjoint1/1
  Ree/1 -> Adjoint/2
  Split Pose/2 -> Terminator1/1
  Gain2/1 -> Adjoint/1
  Sum/1 -> Subsystem/1(u)
  Adjoint1/1 -> Sum/1
  Visual Pursuit Control/5 -> Split Pose/1
  gcheck/1 -> Rate Transition/1
  Switched GP/3(psi) -> out.psi_est/1
  Rate Transition/1 -> Switched GP/1(x)
  Switched GP/2(cov) -> out.GPvarfull/1
  use_GP/1 -> Switch/2
  Switched GP/1(mu) -> Switch/1
  Constant/1 -> Switch/3
  Switch/1 -> Gain2/1

== system unityVPC/Standard VPC/Subsystem ==
  u : Inport
  g : Inport  Port=2
  Adjoint : simlib_vpc_basic/Adjoint  adjointtype=pose
      settings: SourceProductName=VPC Library
  Gain : Gain  Gain=-1
  y : Outport
  wires:
  Adjoint/1 -> y/1
  u/1 -> Gain/1
  g/1 -> Adjoint/2
  Gain/1 -> Adjoint/1

== system unityVPC/VPC + fullGP/Subsystem ==
  u : Inport
  g : Inport  Port=2
  Adjoint : simlib_vpc_basic/Adjoint  adjointtype=pose
      settings: SourceProductName=VPC Library
  Gain : Gain  Gain=-1
  y : Outport
  wires:
  Adjoint/1 -> y/1
  u/1 -> Gain/1
  g/1 -> Adjoint/2
  Gain/1 -> Adjoint/1

== system unityVPC/VPC + switchedGP/Subsystem ==
  u : Inport
  g : Inport  Port=2
  Adjoint : simlib_vpc_basic/Adjoint  adjointtype=pose
      settings: SourceProductName=VPC Library
  Gain : Gain  Gain=-1
  y : Outport
  wires:
  Adjoint/1 -> y/1
  u/1 -> Gain/1
  g/1 -> Adjoint/2
  Gain/1 -> Adjoint/1

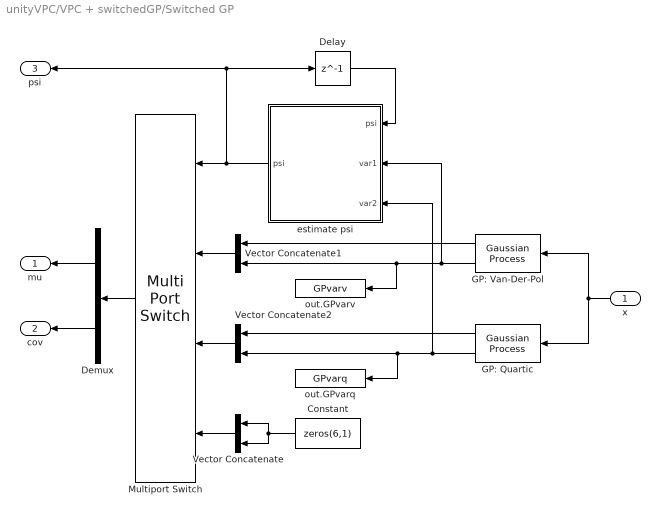
== system unityVPC/VPC + switchedGP/Switched GP ==
  x : Inport
  Constant : Constant  Value=zeros(6,1)
  Delay : Delay  DelayLength=1
  Demux : Demux  Outputs=2
  GP: Quartic : simlib_vpc_gp/Gaussian Process  X=X2  Y=Y2  sigman=sn2  kernel=Squared Exponential ARD  hyp=hyp2
      settings: SourceProductName=VPC Library
  GP: Van-Der-Pol : simlib_vpc_gp/Gaussian Process  X=X1  Y=Y1  sigman=sn1  kernel=Squared Exponential ARD  hyp=hyp1
      settings: SourceProductName=VPC Library
  Multiport Switch : MultiPortSwitch  Inputs=2  DataPortForDefault=Additional data port
  Vector Concatenate : Concatenate
  Vector Concatenate1 : Concatenate
  Vector Concatenate2 : Concatenate
  estimate psi : MATLAB Function  TreatAsAtomicUnit=on
  out.GPvarq : ToWorkspace  VariableName=GPvarq  SaveFormat=Structure With Time  SampleTime=-1
  out.GPvarv : ToWorkspace  VariableName=GPvarv  SaveFormat=Structure With Time  SampleTime=-1
  mu : Outport
  cov : Outport  Port=2
  psi : Outport  Port=3
  wires:
  Constant/1 -> Vector Concatenate/2, Vector Concatenate/1
  Vector Concatenate/1 -> Multiport Switch/4
  Vector Concatenate1/1 -> Multiport Switch/2
  Multiport Switch/1 -> Demux/1
  Vector Concatenate2/1 -> Multiport Switch/3
  GP: Quartic/1 -> Vector Concatenate2/1
  GP: Van-Der-Pol/1 -> Vector Concatenate1/1
  GP: Quartic/2 -> estimate psi/3(var2), out.GPvarq/1, Vector Concatenate2/2
  GP: Van-Der-Pol/2 -> estimate psi/2(var1), out.GPvarv/1, Vector Concatenate1/2
  Demux/1 -> mu/1
  Demux/2 -> cov/1
  x/1 -> GP: Quartic/1, GP: Van-Der-Pol/1
  estimate psi/1(psi) -> psi/1, Delay/1, Multiport Switch/1
  Delay/1 -> estimate psi/1("psi ")

== matlab function unityVPC/VPC + switchedGP/Switched GP/estimate psi ==
  data: psi input; var1 input; psi output; var2 input; var_max parameter; T parameter; alpha parameter
function psi = estim_psi(psi,var1,var2,var_max,T, alpha)
%%ESTIM_PSI estimates the switching signal s(t)
%
% Editor:
%   OMAINSKA Marco - Doctoral Student, Cybernetics
%       <marcoomainska@g.ecc.u-tokyo.ac.jp>
% Review:
%   YAMAUCHI Junya - Assistant Professor
%       <junya_yamauchi@ipc.i.u-tokyo.ac.jp>
%
% Property of: Fujita-Yamauchi Lab, University of Tokyo, 2021
% e-mail: marcoomainska@g.ecc.u-tokyo.ac.jp
% Website: https://www.scl.ipc.i.u-tokyo.ac.jp
% February 2022
%
%------------- BEGIN CODE --------------

% calculate norms
var_norm = zeros(2,1);
var_norm(1) = norm(dot(alpha,var1),2)/var_max(1);
var_norm(2) = norm(dot(alpha,var2),2)/var_max(2);

% estimate switching
if psi == 0 % init case: psi is zero
    [~,psi] = min(var_norm); % find the smallest ||var||/var_max
else
    [~,psi_new] = min(var_norm); % find the smallest ||var||/var_max
    if var_norm(psi) > var_norm(psi_new) + T
        psi = psi_new;
    end
end

% fail safe case
if isnan(psi)
    psi = 0;
end

%-------------- END CODE ---------------
end
